simulink model "SystemModel"  (R2026a)
settings: Solver=FixedStepDiscrete  StopTime=inf  FixedStep=ts_system  EnableMultiTasking=on
StartFcn:
  | Simulink.sdi.setRecordData(false);
undefined symbols (not defined in the file): Battery, BCE12, BCE_Set_init, BMS_Controller_State, Cell10_P, Cell11_P, Cell12_P, Cell1_N, Cell1_P, Cell2_P, Cell3_P, Cell4_P, Cell5_P, Cell6_P, Cell7_P, Cell8_P, Cell9_P, Cell_Temperatures, Cell_Voltages, Charging_State, currentFactor, CV_Gain, Device_01, DiscIntNeverNeededParam, I_cc, MaxCellVoltThrsld, noCurrent, Ns_Module, NumModules, OverCellVoltageLimit, sg_bce, SOCInit, SRE, ts_controller, ts_system, UnderCellVoltageLimit, voltThreshold
libraries: slrealtimeethercatlib x99, fl_lib x65, nesl_utility x43, simulink x23, slrealtimeutilitieslib x13, sl_discontinuities x13, dspstat3 x12, canmsglib x11, speedgoatlib_IO611 x9, batt_lib x3, sharedTrackingLibrary x2, BatteryModuleLibrary_12Cells_lib x1
(part 4 of 6)

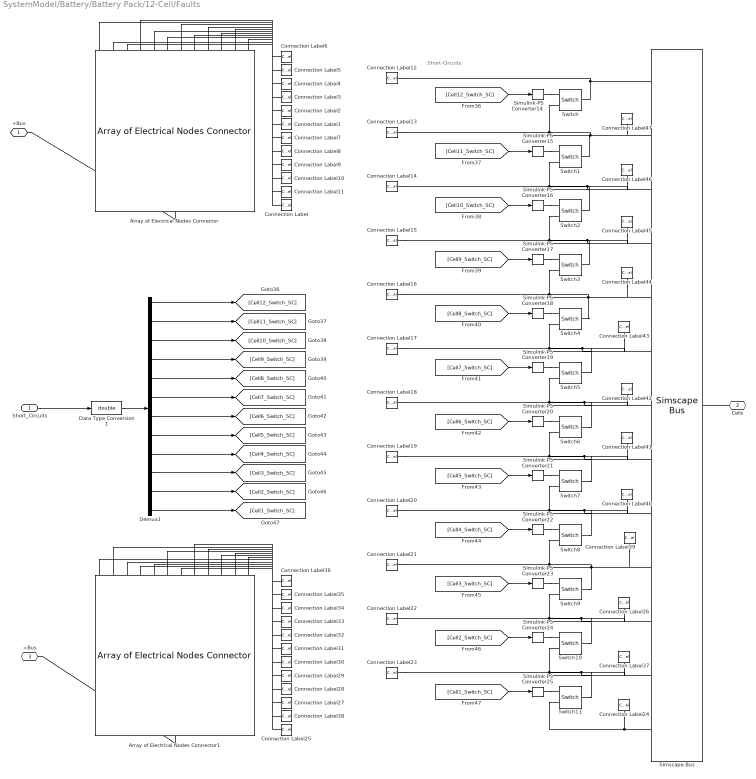
== system SystemModel/Battery/Battery Pack/12-Cell/Faults ==
  note: Short-Circuits
  Short_Circuits : Inport
  Array of Electrical Nodes Connector : batt_lib/Connectors/Array of Electrical Nodes Connector  numInputConnections=simscape.battery.enum.thermal.numArrayOfNodesConnections.twelve  inNode1NumElements=1  inNode2NumElements=1  inNode3NumElements=1  inNode4NumElements=1  inNode5NumElements=1  inNode6NumElements=1  inNode7NumElements=1  inNode8NumElements=1  inNode9NumElements=1  inNode10NumElements=1  inNode11NumElements=1  inNode12NumElements=1  inNode13NumElements=1  inNode14NumElements=1  inNode15NumElements=1  inNode16NumElements=1  inNode17NumElements=1  inNode18NumElements=1  inNode19NumElements=1  inNode20NumElements=1  inNode21NumElements=1  inNode22NumElements=1  inNode23NumElements=1  inNode24NumElements=1  inNode25NumElements=1  inNode26NumElements=1  inNode27NumElements=1  inNode28NumElements=1  inNode29NumElements=1  inNode30NumElements=1  inNode31NumElements=1  inNode32NumElements=1  inNode33NumElements=1  inNode34NumElements=1  inNode35NumElements=1  inNode36NumElements=1  inNode37NumElements=1  inNode38NumElements=1  inNode39NumElements=1  inNode40NumElements=1  inNode41NumElements=1  inNode42NumElements=1  inNode43NumElements=1  inNode44NumElements=1  inNode45NumElements=1  inNode46NumElements=1  inNode47NumElements=1  inNode48NumElements=1  inNode49NumElements=1  inNode50NumElements=1
  Array of Electrical Nodes Connector1 : batt_lib/Connectors/Array of Electrical Nodes Connector  numInputConnections=simscape.battery.enum.thermal.numArrayOfNodesConnections.twelve  inNode1NumElements=1  inNode2NumElements=1  inNode3NumElements=1  inNode4NumElements=1  inNode5NumElements=1  inNode6NumElements=1  inNode7NumElements=1  inNode8NumElements=1  inNode9NumElements=1  inNode10NumElements=1  inNode11NumElements=1  inNode12NumElements=1  inNode13NumElements=1  inNode14NumElements=1  inNode15NumElements=1  inNode16NumElements=1  inNode17NumElements=1  inNode18NumElements=1  inNode19NumElements=1  inNode20NumElements=1  inNode21NumElements=1  inNode22NumElements=1  inNode23NumElements=1  inNode24NumElements=1  inNode25NumElements=1  inNode26NumElements=1  inNode27NumElements=1  inNode28NumElements=1  inNode29NumElements=1  inNode30NumElements=1  inNode31NumElements=1  inNode32NumElements=1  inNode33NumElements=1  inNode34NumElements=1  inNode35NumElements=1  inNode36NumElements=1  inNode37NumElements=1  inNode38NumElements=1  inNode39NumElements=1  inNode40NumElements=1  inNode41NumElements=1  inNode42NumElements=1  inNode43NumElements=1  inNode44NumElements=1  inNode45NumElements=1  inNode46NumElements=1  inNode47NumElements=1  inNode48NumElements=1  inNode49NumElements=1  inNode50NumElements=1
  Connection Label : ConnectionLabel  Label=pos1
  Connection Label1 : ConnectionLabel  Label=pos7
  Connection Label10 : ConnectionLabel  Label=pos3
  Connection Label11 : ConnectionLabel  Label=pos2
  Connection Label12 : ConnectionLabel  Label=pos12
  Connection Label13 : ConnectionLabel  Label=pos11
  Connection Label14 : ConnectionLabel  Label=pos10
  Connection Label15 : ConnectionLabel  Label=pos9
  Connection Label16 : ConnectionLabel  Label=pos8
  Connection Label17 : ConnectionLabel  Label=pos7
  Connection Label18 : ConnectionLabel  Label=pos6
  Connection Label19 : ConnectionLabel  Label=pos5
  Connection Label2 : ConnectionLabel  Label=pos8
  Connection Label20 : ConnectionLabel  Label=pos4
  Connection Label21 : ConnectionLabel  Label=pos3
  Connection Label22 : ConnectionLabel  Label=pos2
  Connection Label23 : ConnectionLabel  Label=pos1
  Connection Label24 : ConnectionLabel  Label=neg1
  Connection Label25 : ConnectionLabel  Label=neg1
  Connection Label26 : ConnectionLabel  Label=neg3
  Connection Label27 : ConnectionLabel  Label=neg3
  Connection Label28 : ConnectionLabel  Label=neg4
  Connection Label29 : ConnectionLabel  Label=neg5
  Connection Label3 : ConnectionLabel  Label=pos9
  Connection Label30 : ConnectionLabel  Label=neg6
  Connection Label31 : ConnectionLabel  Label=neg7
  Connection Label32 : ConnectionLabel  Label=neg8
  Connection Label33 : ConnectionLabel  Label=neg9
  Connection Label34 : ConnectionLabel  Label=neg10
  Connection Label35 : ConnectionLabel  Label=neg11
  Connection Label36 : ConnectionLabel  Label=neg12
  Connection Label37 : ConnectionLabel  Label=neg2
  Connection Label38 : ConnectionLabel  Label=neg2
  Connection Label39 : ConnectionLabel  Label=neg4
  Connection Label4 : ConnectionLabel  Label=pos10
  Connection Label40 : ConnectionLabel  Label=neg5
  Connection Label41 : ConnectionLabel  Label=neg6
  Connection Label42 : ConnectionLabel  Label=neg7
  Connection Label43 : ConnectionLabel  Label=neg8
  Connection Label44 : ConnectionLabel  Label=neg9
  Connection Label45 : ConnectionLabel  Label=neg10
  Connection Label46 : ConnectionLabel  Label=neg11
  Connection Label47 : ConnectionLabel  Label=neg12
  Connection Label5 : ConnectionLabel  Label=pos11
  Connection Label6 : ConnectionLabel  Label=pos12
  Connection Label7 : ConnectionLabel  Label=pos6
  Connection Label8 : ConnectionLabel  Label=pos5
  Connection Label9 : ConnectionLabel  Label=pos4
  Data Type Conversion1 : DataTypeConversion  OutDataTypeStr=double  SaturateOnIntegerOverflow=off  RndMeth=Floor
  Demux1 : Demux  Outputs=12
  Simscape Bus : SimscapeBus  HierarchyStrings=Cell12_P;Cell11_P;Cell10_P;Cell9_P;Cell8_P;Cell7_P;Cell6_P;Cell5_P;Cell4_P;Cell3_P;Cell2_P;Cell1_P;Cell1_N
  Simulink-PS Converter{14..25} (12 alike) : nesl_utility/Simulink-PS Converter  PhysicalDomain=network_engine_domain  SubClassName=ps_input  LeftPortType=input  RightPortType=output  PseudoPeriodic=off  Frequencies=[]  NoiseDistribution=none  NoiseParameters=[]  Unit=1  AffineConversion=off  FilteringAndDerivatives=zero  SimscapeFilterOrder=1  InputFilterTimeConstant=0.001  UdotUserProvided=1
  Switch{,1..11} (12 alike) : fl_lib/Electrical/Electrical Elements/Switch  R_closed=0.01 Ohm  G_open=1e-8 1/Ohm  Threshold=0.5  i_specify=off  i_priority=None  i=0 A  i_nominal_specify=off  i_nominal_value=1  i_nominal_unit=A  v_specify=off  v_priority=None  v=0 V  v_nominal_specify=off  v_nominal_value=1  v_nominal_unit=V
  +Bus : PMIOPort  Side=Right
  Cells : PMIOPort  Port=2  Side=Right
  =Bus : PMIOPort  Port=3  Side=Right
  wires:
  [Cell2_Switch_SC] -> Simulink-PS Converter24/1
  [Cell3_Switch_SC] -> Simulink-PS Converter23/1
  Demux1/9 -> [Cell4_Switch_SC]
  Data Type Conversion1/1 -> Demux1/1
  Demux1/5 -> [Cell8_Switch_SC]
  Demux1/8 -> [Cell5_Switch_SC]
  [Cell1_Switch_SC] -> Simulink-PS Converter25/1
  [Cell12_Switch_SC] -> Simulink-PS Converter14/1
  [Cell11_Switch_SC] -> Simulink-PS Converter15/1
  Demux1/1 -> [Cell12_Switch_SC]
  Demux1/7 -> [Cell6_Switch_SC]
  [Cell4_Switch_SC] -> Simulink-PS Converter22/1
  Demux1/10 -> [Cell3_Switch_SC]
  Demux1/2 -> [Cell11_Switch_SC]
  [Cell8_Switch_SC] -> Simulink-PS Converter18/1
  [Cell5_Switch_SC] -> Simulink-PS Converter21/1
  Demux1/12 -> [Cell1_Switch_SC]
  [Cell10_Switch_SC] -> Simulink-PS Converter16/1
  [Cell9_Switch_SC] -> Simulink-PS Converter17/1
  Demux1/3 -> [Cell10_Switch_SC]
  Demux1/6 -> [Cell7_Switch_SC]
  [Cell6_Switch_SC] -> Simulink-PS Converter20/1
  [Cell7_Switch_SC] -> Simulink-PS Converter19/1
  Demux1/4 -> [Cell9_Switch_SC]
  Demux1/11 -> [Cell2_Switch_SC]
  Short_Circuits/1 -> Data Type Conversion1/1
  connections:
  Simulink-PS Converter17/RConn1 -- Switch3/RConn1
  Connection Label10/LConn1 -- Array of Electrical Nodes Connector/LConn10
  Switch3/LConn1 -- Connection Label45/LConn1 -- Simscape Bus/LConn4 -- Connection Label15/LConn1 -- Switch2/RConn2
  Switch6/LConn1 -- Connection Label42/LConn1 -- Simscape Bus/LConn7 -- Connection Label18/LConn1 -- Switch5/RConn2
  Connection Label31/LConn1 -- Array of Electrical Nodes Connector1/LConn6
  Switch7/LConn1 -- Connection Label41/LConn1 -- Simscape Bus/LConn8 -- Connection Label19/LConn1 -- Switch6/RConn2
  Switch2/LConn1 -- Connection Label46/LConn1 -- Simscape Bus/LConn3 -- Connection Label14/LConn1 -- Switch1/RConn2
  Connection Label28/LConn1 -- Array of Electrical Nodes Connector1/LConn9
  Connection Label29/LConn1 -- Array of Electrical Nodes Connector1/LConn8
  Simulink-PS Converter16/RConn1 -- Switch2/RConn1
  Simulink-PS Converter19/RConn1 -- Switch5/RConn1
  Switch10/LConn1 -- Connection Label26/LConn1 -- Simscape Bus/LConn11 -- Connection Label22/LConn1 -- Switch9/RConn2
  Simulink-PS Converter25/RConn1 -- Switch11/RConn1
  Connection Label27/LConn1 -- Array of Electrical Nodes Connector1/LConn10
  Connection Label25/LConn1 -- Array of Electrical Nodes Connector1/LConn12
  Switch11/LConn1 -- Connection Label37/LConn1 -- Simscape Bus/LConn12 -- Connection Label23/LConn1 -- Switch10/RConn2
  Connection Label39/LConn1 -- Simscape Bus/LConn10 -- Switch9/LConn1 -- Connection Label21/LConn1 -- Switch8/RConn2
  Connection Label36/LConn1 -- Array of Electrical Nodes Connector1/LConn1
  Connection Label34/LConn1 -- Array of Electrical Nodes Connector1/LConn3
  Connection Label35/LConn1 -- Array of Electrical Nodes Connector1/LConn2
  Simulink-PS Converter14/RConn1 -- Switch/RConn1
  Simscape Bus/LConn13 -- Connection Label24/LConn1 -- Switch11/RConn2
  Connection Label30/LConn1 -- Array of Electrical Nodes Connector1/LConn7
  Simulink-PS Converter18/RConn1 -- Switch4/RConn1
  Connection Label44/LConn1 -- Simscape Bus/LConn5 -- Switch4/LConn1 -- Connection Label16/LConn1 -- Switch3/RConn2
  Simulink-PS Converter24/RConn1 -- Switch10/RConn1
  Connection Label33/LConn1 -- Array of Electrical Nodes Connector1/LConn4
  Connection Label38/LConn1 -- Array of Electrical Nodes Connector1/LConn11
  Connection Label32/LConn1 -- Array of Electrical Nodes Connector1/LConn5
  Switch8/LConn1 -- Connection Label40/LConn1 -- Simscape Bus/LConn9 -- Connection Label20/LConn1 -- Switch7/RConn2
  Cells/RConn1 -- Simscape Bus/RConn1
  Simulink-PS Converter20/RConn1 -- Switch6/RConn1
  Simulink-PS Converter15/RConn1 -- Switch1/RConn1
  Simulink-PS Converter21/RConn1 -- Switch7/RConn1
  Simulink-PS Converter23/RConn1 -- Switch9/RConn1
  Simulink-PS Converter22/RConn1 -- Switch8/RConn1
  Connection Label11/LConn1 -- Array of Electrical Nodes Connector/LConn11
  Connection Label6/LConn1 -- Array of Electrical Nodes Connector/LConn1
  Connection Label7/LConn1 -- Array of Electrical Nodes Connector/LConn7
  Switch5/LConn1 -- Connection Label43/LConn1 -- Simscape Bus/LConn6 -- Connection Label17/LConn1 -- Switch4/RConn2
  Connection Label2/LConn1 -- Array of Electrical Nodes Connector/LConn5
  Simscape Bus/LConn1 -- Connection Label12/LConn1 -- Switch/LConn1
  Connection Label4/LConn1 -- Array of Electrical Nodes Connector/LConn3
  Connection Label8/LConn1 -- Array of Electrical Nodes Connector/LConn8
  Connection Label5/LConn1 -- Array of Electrical Nodes Connector/LConn2
  Connection Label3/LConn1 -- Array of Electrical Nodes Connector/LConn4
  Connection Label1/LConn1 -- Array of Electrical Nodes Connector/LConn6
  Connection Label/LConn1 -- Array of Electrical Nodes Connector/LConn12
  Connection Label9/LConn1 -- Array of Electrical Nodes Connector/LConn9
  Connection Label47/LConn1 -- Simscape Bus/LConn2 -- Switch1/LConn1 -- Connection Label13/LConn1 -- Switch/RConn2
  Array of Electrical Nodes Connector1/RConn1 -- =Bus/RConn1
  Array of Electrical Nodes Connector/RConn1 -- +Bus/RConn1

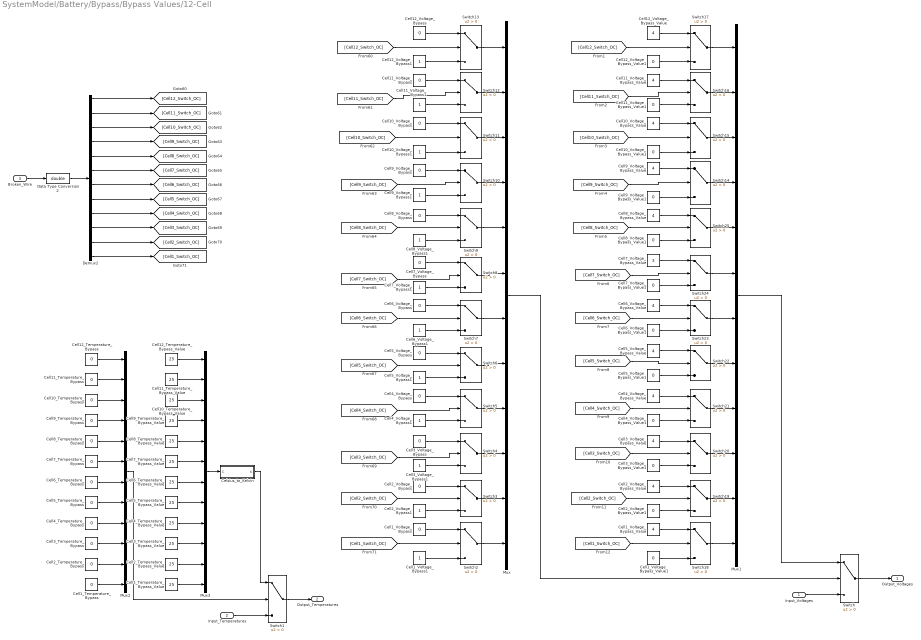
== system SystemModel/Battery/Bypass/Bypass Values/12-Cell ==
  Input_Voltages : Inport
  Input_Temperatures : Inport  Port=2
  Broken_Wire : Inport  Port=3
  Cell10_Temperature_Bypass : Constant  Value=0  SampleTime=-1
  Cell10_Temperature_Bypass_Value : Constant  Value=25  SampleTime=-1
  Cell10_Voltage_Bypass : Constant  Value=0  SampleTime=-1
  Cell10_Voltage_Bypass1 : Constant  SampleTime=-1
  Cell10_Voltage_Bypass_Value : Constant  Value=4  SampleTime=-1
  Cell10_Voltage_Bypass_Value1 : Constant  Value=0  SampleTime=-1
  Cell11_Temperature_Bypass : Constant  Value=0  SampleTime=-1
  Cell11_Temperature_Bypass_Value : Constant  Value=25  SampleTime=-1
  Cell11_Voltage_Bypass : Constant  Value=0  SampleTime=-1
  Cell11_Voltage_Bypass1 : Constant  SampleTime=-1
  Cell11_Voltage_Bypass_Value : Constant  Value=4  SampleTime=-1
  Cell11_Voltage_Bypass_Value1 : Constant  Value=0  SampleTime=-1
  Cell12_Temperature_Bypass : Constant  Value=0  SampleTime=-1
  Cell12_Temperature_Bypass_Value : Constant  Value=25  SampleTime=-1
  Cell12_Voltage_Bypass : Constant  Value=0  SampleTime=-1
  Cell12_Voltage_Bypass1 : Constant  SampleTime=-1
  Cell12_Voltage_Bypass_Value : Constant  Value=4  SampleTime=-1
  Cell12_Voltage_Bypass_Value1 : Constant  Value=0  SampleTime=-1
  Cell1_Temperature_Bypass : Constant  Value=0  SampleTime=-1
  Cell1_Temperature_Bypass_Value : Constant  Value=25  SampleTime=-1
  Cell1_Voltage_Bypass : Constant  Value=0  SampleTime=-1
  Cell1_Voltage_Bypass1 : Constant  SampleTime=-1
  Cell1_Voltage_Bypass_Value : Constant  Value=4  SampleTime=-1
  Cell1_Voltage_Bypass_Value1 : Constant  Value=0  SampleTime=-1
  Cell2_Temperature_Bypass : Constant  Value=0  SampleTime=-1
  Cell2_Temperature_Bypass_Value : Constant  Value=25  SampleTime=-1
  Cell2_Voltage_Bypass : Constant  Value=0  SampleTime=-1
  Cell2_Voltage_Bypass1 : Constant  SampleTime=-1
  Cell2_Voltage_Bypass_Value : Constant  Value=4  SampleTime=-1
  Cell2_Voltage_Bypass_Value1 : Constant  Value=0  SampleTime=-1
  Cell3_Temperature_Bypass : Constant  Value=0  SampleTime=-1
  Cell3_Temperature_Bypass_Value : Constant  Value=25  SampleTime=-1
  Cell3_Voltage_Bypass : Constant  Value=0  SampleTime=-1
  Cell3_Voltage_Bypass1 : Constant  SampleTime=-1
  Cell3_Voltage_Bypass_Value : Constant  Value=4  SampleTime=-1
  Cell3_Voltage_Bypass_Value1 : Constant  Value=0  SampleTime=-1
  Cell4_Temperature_Bypass : Constant  Value=0  SampleTime=-1
  Cell4_Temperature_Bypass_Value : Constant  Value=25  SampleTime=-1
  Cell4_Voltage_Bypass : Constant  Value=0  SampleTime=-1
  Cell4_Voltage_Bypass1 : Constant  SampleTime=-1
  Cell4_Voltage_Bypass_Value : Constant  Value=4  SampleTime=-1
  Cell4_Voltage_Bypass_Value1 : Constant  Value=0  SampleTime=-1
  Cell5_Temperature_Bypass : Constant  Value=0  SampleTime=-1
  Cell5_Temperature_Bypass_Value : Constant  Value=25  SampleTime=-1
  Cell5_Voltage_Bypass : Constant  Value=0  SampleTime=-1
  Cell5_Voltage_Bypass1 : Constant  SampleTime=-1
  Cell5_Voltage_Bypass_Value : Constant  Value=4  SampleTime=-1
  Cell5_Voltage_Bypass_Value1 : Constant  Value=0  SampleTime=-1
  Cell6_Temperature_Bypass : Constant  Value=0  SampleTime=-1
  Cell6_Temperature_Bypass_Value : Constant  Value=25  SampleTime=-1
  Cell6_Voltage_Bypass : Constant  Value=0  SampleTime=-1
  Cell6_Voltage_Bypass1 : Constant  SampleTime=-1
  Cell6_Voltage_Bypass_Value : Constant  Value=4  SampleTime=-1
  Cell6_Voltage_Bypass_Value1 : Constant  Value=0  SampleTime=-1
  Cell7_Temperature_Bypass : Constant  Value=0  SampleTime=-1
  Cell7_Temperature_Bypass_Value : Constant  Value=25  SampleTime=-1
  Cell7_Voltage_Bypass : Constant  Value=0  SampleTime=-1
  Cell7_Voltage_Bypass1 : Constant  SampleTime=-1
  Cell7_Voltage_Bypass_Value : Constant  Value=3  SampleTime=-1
  Cell7_Voltage_Bypass_Value1 : Constant  Value=0  SampleTime=-1
  Cell8_Temperature_Bypass : Constant  Value=0  SampleTime=-1
  Cell8_Temperature_Bypass_Value : Constant  Value=25  SampleTime=-1
  Cell8_Voltage_Bypass : Constant  Value=0  SampleTime=-1
  Cell8_Voltage_Bypass1 : Constant  SampleTime=-1
  Cell8_Voltage_Bypass_Value : Constant  Value=4  SampleTime=-1
  Cell8_Voltage_Bypass_Value1 : Constant  Value=0  SampleTime=-1
  Cell9_Temperature_Bypass : Constant  Value=0  SampleTime=-1
  Cell9_Temperature_Bypass_Value : Constant  Value=25  SampleTime=-1
  Cell9_Voltage_Bypass : Constant  Value=0  SampleTime=-1
  Cell9_Voltage_Bypass1 : Constant  SampleTime=-1
  Cell9_Voltage_Bypass_Value : Constant  Value=4  SampleTime=-1
  Cell9_Voltage_Bypass_Value1 : Constant  Value=0  SampleTime=-1
  Celsius_to_Kelvin : Subsystem
  Data Type Conversion2 : DataTypeConversion  OutDataTypeStr=double  SaturateOnIntegerOverflow=off  RndMeth=Floor
  Demux2 : Demux  Outputs=12
  Mux{,1..3} (4 alike) : Mux  Inputs=12
  Switch{,1..25} (26 alike) : Switch  Criteria=u2 > Threshold  SaturateOnIntegerOverflow=off  InputSameDT=off
  Output_Voltages : Outport
  Output_Temperatures : Outport  Port=2
  wires:
  Mux/1 -> Switch/2
  Switch/1 -> Output_Voltages/1
  Mux1/1 -> Switch/1
  Input_Voltages/1 -> Switch/3
  Cell11_Temperature_Bypass/1 -> Mux2/2
  Cell1_Temperature_Bypass/1 -> Mux2/12
  Cell5_Temperature_Bypass/1 -> Mux2/8
  Cell6_Temperature_Bypass/1 -> Mux2/7
  Cell10_Temperature_Bypass/1 -> Mux2/3
  Cell4_Temperature_Bypass/1 -> Mux2/9
  Cell2_Temperature_Bypass/1 -> Mux2/11
  Cell9_Temperature_Bypass/1 -> Mux2/4
  Cell8_Temperature_Bypass_Value/1 -> Mux3/5
  Cell10_Temperature_Bypass_Value/1 -> Mux3/3
  Mux3/1 -> Celsius_to_Kelvin/1(C)
  Cell12_Temperature_Bypass_Value/1 -> Mux3/1
  Cell1_Temperature_Bypass_Value/1 -> Mux3/12
  Cell11_Temperature_Bypass_Value/1 -> Mux3/2
  Cell8_Temperature_Bypass/1 -> Mux2/5
  Cell3_Temperature_Bypass_Value/1 -> Mux3/10
  Cell9_Temperature_Bypass_Value/1 -> Mux3/4
  Cell6_Temperature_Bypass_Value/1 -> Mux3/7
  Cell12_Temperature_Bypass/1 -> Mux2/1
  Cell5_Temperature_Bypass_Value/1 -> Mux3/8
  Cell2_Temperature_Bypass_Value/1 -> Mux3/11
  Cell7_Temperature_Bypass/1 -> Mux2/6
  Mux2/1 -> Switch1/2
  Celsius_to_Kelvin/1(K) -> Switch1/1
  Cell4_Temperature_Bypass_Value/1 -> Mux3/9
  Input_Temperatures/1 -> Switch1/3
  Cell3_Temperature_Bypass/1 -> Mux2/10
  Cell7_Temperature_Bypass_Value/1 -> Mux3/6
  Switch1/1 -> Output_Temperatures/1
  Switch2/1 -> Mux/12
  [Cell5_Switch_OC] -> Switch6/2
  [Cell1_Switch_OC] -> Switch2/2
  [Cell8_Switch_OC] -> Switch9/2
  [Cell6_Switch_OC] -> Switch7/2
  [Cell7_Switch_OC] -> Switch8/2
  [Cell10_Switch_OC] -> Switch11/2
  [Cell12_Switch_OC] -> Switch13/2
  [Cell3_Switch_OC] -> Switch4/2
  [Cell9_Switch_OC] -> Switch10/2
  [Cell4_Switch_OC] -> Switch5/2
  [Cell11_Switch_OC] -> Switch12/2
  [Cell2_Switch_OC] -> Switch3/2
  Switch3/1 -> Mux/11
  Switch13/1 -> Mux/1
  Switch12/1 -> Mux/2
  Switch11/1 -> Mux/3
  Switch10/1 -> Mux/4
  Switch9/1 -> Mux/5
  Switch8/1 -> Mux/6
  Switch7/1 -> Mux/7
  Switch6/1 -> Mux/8
  Switch5/1 -> Mux/9
  Switch4/1 -> Mux/10
  Cell1_Voltage_Bypass/1 -> Switch2/1
  Cell2_Voltage_Bypass/1 -> Switch3/1
  Cell12_Voltage_Bypass/1 -> Switch13/1
  Cell11_Voltage_Bypass/1 -> Switch12/1
  Cell10_Voltage_Bypass/1 -> Switch11/1
  Cell9_Voltage_Bypass/1 -> Switch10/1
  Cell8_Voltage_Bypass/1 -> Switch9/1
  Cell7_Voltage_Bypass/1 -> Switch8/1
  Cell6_Voltage_Bypass/1 -> Switch7/1
  Cell5_Voltage_Bypass/1 -> Switch6/1
  Cell4_Voltage_Bypass/1 -> Switch5/1
  Cell3_Voltage_Bypass/1 -> Switch4/1
  Cell1_Voltage_Bypass1/1 -> Switch2/3
  Cell2_Voltage_Bypass1/1 -> Switch3/3
  Cell3_Voltage_Bypass1/1 -> Switch4/3
  Cell4_Voltage_Bypass1/1 -> Switch5/3
  Cell5_Voltage_Bypass1/1 -> Switch6/3
  Cell6_Voltage_Bypass1/1 -> Switch7/3
  Cell7_Voltage_Bypass1/1 -> Switch8/3
  Cell8_Voltage_Bypass1/1 -> Switch9/3
  Cell9_Voltage_Bypass1/1 -> Switch10/3
  Cell10_Voltage_Bypass1/1 -> Switch11/3
  Cell11_Voltage_Bypass1/1 -> Switch12/3
  Cell12_Voltage_Bypass1/1 -> Switch13/3
  Switch17/1 -> Mux1/1
  Switch16/1 -> Mux1/2
  Switch18/1 -> Mux1/12
  Switch25/1 -> Mux1/5
  Switch20/1 -> Mux1/10
  Switch19/1 -> Mux1/11
  Switch15/1 -> Mux1/3
  Switch14/1 -> Mux1/4
  Switch24/1 -> Mux1/6
  Switch23/1 -> Mux1/7
  Switch22/1 -> Mux1/8
  Switch21/1 -> Mux1/9
  Cell12_Voltage_Bypass_Value/1 -> Switch17/1
  Cell11_Voltage_Bypass_Value/1 -> Switch16/1
  Cell10_Voltage_Bypass_Value/1 -> Switch15/1
  Cell9_Voltage_Bypass_Value/1 -> Switch14/1
  Cell8_Voltage_Bypass_Value/1 -> Switch25/1
  Cell6_Voltage_Bypass_Value/1 -> Switch23/1
  Cell5_Voltage_Bypass_Value/1 -> Switch22/1
  Cell4_Voltage_Bypass_Value/1 -> Switch21/1
  Cell3_Voltage_Bypass_Value/1 -> Switch20/1
  Cell2_Voltage_Bypass_Value/1 -> Switch19/1
  Cell1_Voltage_Bypass_Value/1 -> Switch18/1
  Cell7_Voltage_Bypass_Value/1 -> Switch24/1
  Cell12_Voltage_Bypass_Value1/1 -> Switch17/3
  Cell11_Voltage_Bypass_Value1/1 -> Switch16/3
  Cell10_Voltage_Bypass_Value1/1 -> Switch15/3
  Cell9_Voltage_Bypass_Value1/1 -> Switch14/3
  Cell8_Voltage_Bypass_Value1/1 -> Switch25/3
  Cell7_Voltage_Bypass_Value1/1 -> Switch24/3
  Cell6_Voltage_Bypass_Value1/1 -> Switch23/3
  Cell5_Voltage_Bypass_Value1/1 -> Switch22/3
  Cell4_Voltage_Bypass_Value1/1 -> Switch21/3
  Cell3_Voltage_Bypass_Value1/1 -> Switch20/3
  Cell2_Voltage_Bypass_Value1/1 -> Switch19/3
  Cell1_Voltage_Bypass_Value1/1 -> Switch18/3
  [Cell12_Switch_OC] -> Switch17/2
  [Cell10_Switch_OC] -> Switch15/2
  [Cell11_Switch_OC] -> Switch16/2
  [Cell9_Switch_OC] -> Switch14/2
  [Cell8_Switch_OC] -> Switch25/2
  [Cell7_Switch_OC] -> Switch24/2
  [Cell6_Switch_OC] -> Switch23/2
  [Cell5_Switch_OC] -> Switch22/2
  [Cell4_Switch_OC] -> Switch21/2
  [Cell3_Switch_OC] -> Switch20/2
  [Cell2_Switch_OC] -> Switch19/2
  [Cell1_Switch_OC] -> Switch18/2
  Demux2/6 -> [Cell7_Switch_OC]
  Demux2/12 -> [Cell1_Switch_OC]
  Broken_Wire/1 -> Data Type Conversion2/1
  Demux2/5 -> [Cell8_Switch_OC]
  Demux2/11 -> [Cell2_Switch_OC]
  Demux2/7 -> [Cell6_Switch_OC]
  Demux2/3 -> [Cell10_Switch_OC]
  Demux2/9 -> [Cell4_Switch_OC]
  Demux2/2 -> [Cell11_Switch_OC]
  Demux2/10 -> [Cell3_Switch_OC]
  Demux2/4 -> [Cell9_Switch_OC]
  Demux2/8 -> [Cell5_Switch_OC]
  Data Type Conversion2/1 -> Demux2/1
  Demux2/1 -> [Cell12_Switch_OC]

== system SystemModel/Battery/HW Interface/BCE - HIL/Battery Cell Emulator ==
  Sensor_Values_Sim : Inport
  "BCE Bus Packing " : Subsystem
  "BCE Read " : Subsystem  InitFcn=sg_bce.checkNumberOfBlocksGlobal(bdroot);  mask(bce_read){}
      settings: OpenFcn=sg_bce.openFcnRead;
      mask Help: eval('sg.utils.help.show(''io_main/refentry_bce_read'');')
      mask Display: disp('Speedgoat\nBMTS Read\nEtherCAT Bus: 0, Device: 1\nBCE12-0505');port_label('output',1,'Data');
  "BCE Setup " : Subsystem  LoadFcn=|  InitFcn=|  mask(bce_setup){}
      LoadFcn=|
      | sg_bce.createBusSignals;
      | sg_bce.setupEniCallback(gcb, bdroot);
      InitFcn=|
      | sg_bce.createBusSignals;
      | sg_bce.checkNumberOfBlocksGlobal(bdroot);
      mask init:
      | sg_bce.setupEniCallback(gcb, bdroot);
      settings: OpenFcn=sg_bce.openFcnSetup;
      mask Help: eval('sg.utils.help.show(''io_main/refentry_bce_setup'');')
      mask Display: disp('Speedgoat\nBattery Management Testing Systems\nEtherCAT Bus: 0\nSetup');
  "BCE Write " : Subsystem  InitFcn=sg_bce.checkNumberOfBlocksGlobal(bdroot);  mask(bce_write){}
      settings: OpenFcn=sg_bce.openFcnWrite;
      mask Help: eval('sg.utils.help.show(''io_main/refentry_bce_write'');')
      mask Display: disp('Speedgoat\nBMTS Write\nEtherCAT Bus: 0, Device: 1\nBCE12-0505');port_label('input',1,'Data');
  BCE_Init : Switch  Criteria=u2 > Threshold  SaturateOnIntegerOverflow=off  InputSameDT=off
  Bus Selector : BusSelector  OutputSignals=Cell_12.I,Cell_11.I,Cell_10.I,Cell_9.I,Cell_8.I,Cell_7.I,Cell_6.I,Cell_5.I,Cell_4.I,Cell_3.I,Cell_2.I,Cell_1.I
  Bus Selector1 : BusSelector  OutputSignals=Cell_Voltages
  Bus Selector2 : BusSelector  OutputSignals=Cell_12.V,Cell_11.V,Cell_10.V,Cell_9.V,Cell_8.V,Cell_7.V,Cell_6.V,Cell_5.V,Cell_4.V,Cell_3.V,Cell_2.V,Cell_1.V
  Constant : Constant  Value=[0,0,0,0,0,0,0,0,0,0,0,0]
  Data Type Conversion : DataTypeConversion  OutDataTypeStr=single  SaturateOnIntegerOverflow=off  RndMeth=Floor
  Data Type Conversion1 : DataTypeConversion  OutDataTypeStr=boolean  SaturateOnIntegerOverflow=off  RndMeth=Floor
  Data Type Conversion2 : DataTypeConversion  OutDataTypeStr=single  SaturateOnIntegerOverflow=off  RndMeth=Floor
  Demux : Demux  Outputs=12
  Enable : Constant
  Mux : Mux  Inputs=12
  Mux1 : Mux  Inputs=12
  No_current : Constant  Value=0
  Step : Step  Time=2
  Current_Values : Outport
  Cell_Voltages : Outport  Port=2
  wires:
  Sensor_Values_Sim/1 -> Bus Selector1/1
  BCE_Init/1 -> Demux/1
  "BCE Read "/1(Data) -> Bus Selector/1, Bus Selector2/1
  Constant/1 -> Data Type Conversion2/1
  Step/1 -> BCE_Init/2
  "BCE Bus Packing "/1(BCE Bus) -> "BCE Write "/1(Data)
  No_current/1 -> Data Type Conversion/1
  Data Type Conversion2/1 -> BCE_Init/3
  Bus Selector/1 -> Mux/1  "<I>"
  Bus Selector/2 -> Mux/2  "<I>"
  Bus Selector/3 -> Mux/3  "<I>"
  Bus Selector/4 -> Mux/4  "<I>"
  Bus Selector/5 -> Mux/5  "<I>"
  Bus Selector/6 -> Mux/6  "<I>"
  Bus Selector/7 -> Mux/7  "<I>"
  Bus Selector/8 -> Mux/8  "<I>"
  Bus Selector/9 -> Mux/9  "<I>"
  Bus Selector/10 -> Mux/10  "<I>"
  Bus Selector/11 -> Mux/11  "<I>"
  Bus Selector/12 -> Mux/12  "<I>"
  Mux/1 -> Current_Values/1
  Bus Selector2/1 -> Mux1/1  "<V>"
  Bus Selector2/2 -> Mux1/2  "<V>"
  Bus Selector2/3 -> Mux1/3  "<V>"
  Bus Selector2/4 -> Mux1/4  "<V>"
  Bus Selector2/5 -> Mux1/5  "<V>"
  Bus Selector2/6 -> Mux1/6  "<V>"
  Bus Selector2/7 -> Mux1/7  "<V>"
  Bus Selector2/8 -> Mux1/8  "<V>"
  Bus Selector2/9 -> Mux1/9  "<V>"
  Bus Selector2/10 -> Mux1/10  "<V>"
  Bus Selector2/11 -> Mux1/11  "<V>"
  Bus Selector2/12 -> Mux1/12  "<V>"
  Mux1/1 -> Cell_Voltages/1
  Bus Selector1/1 -> BCE_Init/1  "<Cell_Voltages>"
  Enable/1 -> Data Type Conversion1/1
  Data Type Conversion1/1 -> "BCE Bus Packing "/1(Cell 1 Enable), "BCE Bus Packing "/9(Cell 9 Enable), "BCE Bus Packing "/12(Cell 12 Enable), "BCE Bus Packing "/11(Cell 11 Enable), "BCE Bus Packing "/10(Cell 10 Enable), "BCE Bus Packing "/8(Cell 8 Enable), "BCE Bus Packing "/7(Cell 7 Enable), "BCE Bus Packing "/6(Cell 6 Enable), "BCE Bus Packing "/5(Cell 5 Enable), "BCE Bus Packing "/4(Cell 4 Enable), "BCE Bus Packing "/3(Cell 3 Enable), "BCE Bus Packing "/2(Cell 2 Enable)
  Data Type Conversion/1 -> "BCE Bus Packing "/29(Cell 5 Current), "BCE Bus Packing "/28(Cell 4 Current), "BCE Bus Packing "/25(Cell 1 Current), "BCE Bus Packing "/26(Cell 2 Current), "BCE Bus Packing "/27(Cell 3 Current), "BCE Bus Packing "/30(Cell 6 Current), "BCE Bus Packing "/31(Cell 7 Current), "BCE Bus Packing "/32(Cell 8 Current), "BCE Bus Packing "/33(Cell 9 Current), "BCE Bus Packing "/34(Cell 10 Current), "BCE Bus Packing "/35(Cell 11 Current), "BCE Bus Packing "/36(Cell 12 Current)
  Demux/1 -> "BCE Bus Packing "/13(Cell 12 Voltage)
  Demux/2 -> "BCE Bus Packing "/14(Cell 11 Voltage)
  Demux/3 -> "BCE Bus Packing "/15(Cell 10 Voltage)
  Demux/4 -> "BCE Bus Packing "/16(Cell 9 Voltage)
  Demux/5 -> "BCE Bus Packing "/17(Cell 8 Voltage)
  Demux/6 -> "BCE Bus Packing "/18(Cell 7 Voltage)
  Demux/7 -> "BCE Bus Packing "/19(Cell 6 Voltage)
  Demux/8 -> "BCE Bus Packing "/20(Cell 5 Voltage)
  Demux/9 -> "BCE Bus Packing "/21(Cell 4 Voltage)
  Demux/10 -> "BCE Bus Packing "/22(Cell 3 Voltage)
  Demux/11 -> "BCE Bus Packing "/23(Cell 2 Voltage)
  Demux/12 -> "BCE Bus Packing "/24(Cell 1 Voltage)

== system SystemModel/Battery/HW Interface/BCE - HIL/Shunt Emulator ==
  note: Shunt Emulator Blocks
  Sensor_Values_Sim : Inport
  Bus Selector : BusSelector  OutputSignals=Pack_Current
  Pack_Current : Outport
  wires:
  Sensor_Values_Sim/1 -> Bus Selector/1
  Bus Selector/1 -> Pack_Current/1  "<Pack_Current>"

== system SystemModel/Battery/HW Interface/BCE - HIL/Temperature Emulator ==
  note: Temperature Emulation Blocks
  Sensor_Values_Sim : Inport
  Bus Selector : BusSelector  OutputSignals=Cell_Temperatures
  Cell_Temperatures : Outport
  wires:
  Sensor_Values_Sim/1 -> Bus Selector/1
  Bus Selector/1 -> Cell_Temperatures/1  "<Cell_Temperatures>"

== system SystemModel/Instrumentation/Instrumented Signals/12-Cell/Celsius_to_Kelvin ==
  K : Inport
  Add : Sum  Inputs=+-
  Constant4 : Constant  Value=273.15
  C : Outport
  wires:
  Constant4/1 -> Add/2
  K/1 -> Add/1
  Add/1 -> C/1

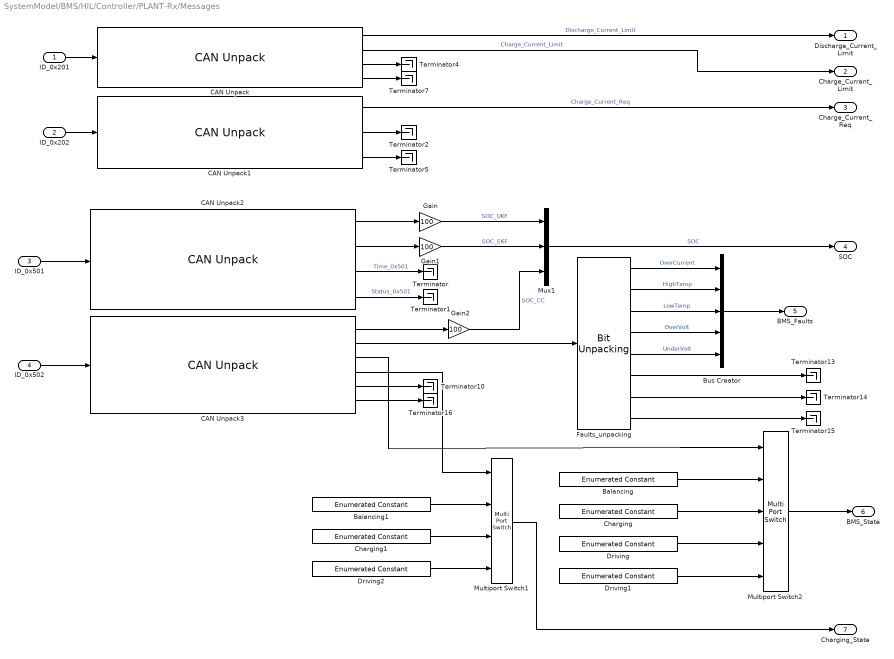
== system SystemModel/BMS/HIL/Controller/PLANT-Rx/Messages ==
  ID_0x201 : Inport
  ID_0x202 : Inport  Port=2
  ID_0x501 : Inport  Port=3
  ID_0x502 : Inport  Port=4
  Balancing : simulink/Sources/Enumerated Constant  OutDataTypeStr=Enum: BMS_Controller_State  Value=BMS_Controller_State.BMS_Idle  SampleTime=-1
  Balancing1 : simulink/Sources/Enumerated Constant  OutDataTypeStr=Enum: Charging_State  Value=Charging_State.Init  SampleTime=-1
  Bus Creator : BusCreator  Inputs=5  OutDataTypeStr=Bus: Faults
  CAN Unpack : canmsglib/CAN Unpack  MsgList=(none)  MsgName=CAN Msg  MsgIDType=Standard (11-bit identifier)  MsgIdentifier=0x201  MsgLength=8  SignalInfo={ 'DischargeCurrentLimit_CAN', '0', '32', 'LE', 'single', 'Standard', '0', '1', '0', '-inf', '+inf'; 'ChargeCurrentLimit_CAN', '32', '32', 'LE', 'single', 'Standard', '0', '1', '0', '-Inf', 'Inf' }  IDPort=off  TimestampPort=on  ErrorPort=off  RemotePort=off  LengthPort=off  StatusPort=on  ApplyMinMax=off
      settings: LibrarySourceBlock=embeddedtargetslib/Host Communication/CAN Unpack
  CAN Unpack1 : canmsglib/CAN Unpack  MsgList=(none)  MsgName=CAN Msg  MsgIDType=Standard (11-bit identifier)  MsgIdentifier=0x202  MsgLength=4  SignalInfo={ 'ChargeCurrentReq', '0', '32', 'LE', 'single', 'Standard', '0', '1', '0', '-inf', '+inf' }  IDPort=off  TimestampPort=on  ErrorPort=off  RemotePort=off  LengthPort=off  StatusPort=on  ApplyMinMax=off
      settings: LibrarySourceBlock=embeddedtargetslib/Host Communication/CAN Unpack
  CAN Unpack2 : canmsglib/CAN Unpack  MsgList=(none)  MsgName=CAN Msg  MsgIDType=Standard (11-bit identifier)  MsgIdentifier=0x501  MsgLength=8  SignalInfo={ 'SOC_UKF', '0', '32', 'LE', 'single', 'Standard', '0', '1', '0', '-inf', '+inf'; 'SOC_EKF', '32', '32', 'LE', 'single', 'Standard', '0', '1', '0', '-Inf', 'Inf' }  IDPort=off  TimestampPort=on  ErrorPort=off  RemotePort=off  LengthPort=off  StatusPort=on  ApplyMinMax=off
      settings: LibrarySourceBlock=embeddedtargetslib/Host Communication/CAN Unpack
  CAN Unpack3 : canmsglib/CAN Unpack  MsgList=(none)  MsgName=CAN Msg  MsgIDType=Standard (11-bit identifier)  MsgIdentifier=0x502  MsgLength=7  SignalInfo={ 'SOC_CC', '0', '32', 'LE', 'single', 'Standard', '0', '1', '0', '-inf', '+inf'; 'Faults', '32', '8', 'LE', 'unsigned', 'Standard', '0', '1', '0', '-Inf', 'Inf'; 'BMS_State', '40', '8', 'LE', 'unsigned', 'Standard', '0', '1', '0', '-Inf', 'Inf'; 'Charging_State', '48', '8', 'LE', 'signed', 'Standard', '0', '1', '0', '-Inf', 'Inf' }  IDPort=off  TimestampPort=on  ErrorPort=off  RemotePort=off  LengthPort=off  StatusPort=on  ApplyMinMax=off
      settings: LibrarySourceBlock=embeddedtargetslib/Host Communication/CAN Unpack
  Charging : simulink/Sources/Enumerated Constant  OutDataTypeStr=Enum: BMS_Controller_State  Value=BMS_Controller_State.BMS_Driving  SampleTime=-1
  Charging1 : simulink/Sources/Enumerated Constant  OutDataTypeStr=Enum: Charging_State  Value=Charging_State.CC  SampleTime=-1
  Driving : simulink/Sources/Enumerated Constant  OutDataTypeStr=Enum: BMS_Controller_State  Value=BMS_Controller_State.BMS_Charging  SampleTime=-1
  Driving1 : simulink/Sources/Enumerated Constant  OutDataTypeStr=Enum: BMS_Controller_State  Value=BMS_Controller_State.BMS_Fault  SampleTime=-1
  Driving2 : simulink/Sources/Enumerated Constant  OutDataTypeStr=Enum: Charging_State  Value=Charging_State.CV  SampleTime=-1
  Faults_unpacking : slrealtimeutilitieslib/Bit Unpacking  SignExtend=on  MaskBitPatterns={[7:7] [6:6] [5:5] [4:4] [3:3] [2:2] [1:1] [0:0]}  MaskPackDataType=uint8  MaskPackDataSize=[1]  MaskUnpackDataTypes={'boolean', 'boolean', 'boolean', 'boolean', 'boolean', 'boolean', 'boolean', 'boolean'}  MaskUnpackDataSizes={[1] [1] [1] [1] [1] [1] [1] [1]}
  Gain : Gain  Gain=100
  Gain1 : Gain  Gain=100
  Gain2 : Gain  Gain=100
  Multiport Switch1 : MultiPortSwitch  DataPortOrder=Zero-based contiguous  zeroidx=on  SaturateOnIntegerOverflow=off  InputSameDT=off
  Multiport Switch2 : MultiPortSwitch  DataPortOrder=Zero-based contiguous  Inputs=4  zeroidx=on  SaturateOnIntegerOverflow=off  InputSameDT=off
  Mux1 : Mux  Inputs=3
  Terminator{,1..2,4..5,7,10,13..16} (11 alike) : Terminator
  Discharge_Current_Limit : Outport
  Charge_Current_Limit : Outport  Port=2
  Charge_Current_Req : Outport  Port=3
  SOC : Outport  Port=4
  BMS_Faults : Outport  Port=5
  BMS_State : Outport  Port=6
  Charging_State : Outport  Port=7
  wires:
  CAN Unpack1/2 -> Terminator2/1
  CAN Unpack/1 -> Discharge_Current_Limit/1  "Discharge_Current_Limit"
  CAN Unpack1/1 -> Charge_Current_Req/1  "Charge_Current_Req"
  CAN Unpack1/3 -> Terminator5/1
  CAN Unpack/2 -> Charge_Current_Limit/1  "Charge_Current_Limit"
  CAN Unpack/4 -> Terminator7/1
  CAN Unpack/3 -> Terminator4/1
  ID_0x201/1 -> CAN Unpack/1
  ID_0x202/1 -> CAN Unpack1/1
  CAN Unpack2/2 -> Gain1/1
  Bus Creator/1 -> BMS_Faults/1
  Faults_unpacking/5 -> Bus Creator/5  "UnderVolt"
  CAN Unpack3/5 -> Terminator10/1
  CAN Unpack3/3 -> Multiport Switch2/1
  CAN Unpack3/2 -> Faults_unpacking/1
  Faults_unpacking/4 -> Bus Creator/4  "OverVolt"
  Faults_unpacking/3 -> Bus Creator/3  "LowTemp"
  CAN Unpack2/1 -> Gain/1
  Faults_unpacking/1 -> Bus Creator/1  "OverCurrent"
  ID_0x501/1 -> CAN Unpack2/1
  Faults_unpacking/2 -> Bus Creator/2  "HighTemp"
  CAN Unpack2/3 -> Terminator/1  "Time_0x501"
  ID_0x502/1 -> CAN Unpack3/1
  Gain/1 -> Mux1/1  "SOC_UKF"
  Gain1/1 -> Mux1/2  "SOC_EKF"
  CAN Unpack3/1 -> Gain2/1
  CAN Unpack2/4 -> Terminator1/1  "Status_0x501"
  Faults_unpacking/6 -> Terminator13/1
  Faults_unpacking/7 -> Terminator14/1
  Faults_unpacking/8 -> Terminator15/1
  CAN Unpack3/6 -> Terminator16/1
  Gain2/1 -> Mux1/3  "SOC_CC"
  Mux1/1 -> SOC/1  "SOC"
  Charging/1 -> Multiport Switch2/3
  Balancing/1 -> Multiport Switch2/2
  Driving/1 -> Multiport Switch2/4
  Driving1/1 -> Multiport Switch2/5
  Charging1/1 -> Multiport Switch1/3
  Driving2/1 -> Multiport Switch1/4
  Balancing1/1 -> Multiport Switch1/2
  CAN Unpack3/4 -> Multiport Switch1/1
  Multiport Switch1/1 -> Charging_State/1
  Multiport Switch2/1 -> BMS_State/1

== system SystemModel/BMS/HIL/Controller/PLANT-Tx/12-Cell ==
  to_Controller : Inport
  to_Controller_SRE : Inport  Port=2
  Bus Selector : BusSelector  OutputSignals=Pack_Current,Cell_Temperatures
  CAN Pack2 : canmsglib/CAN Pack  MsgList=(none)  MsgName=CAN Msg  MsgIDType=Standard (11-bit identifier)  MsgIdentifier=0x407  CANIDInput=off  MsgLength=8  Remote=off  ApplyMinMax=off  BusOutput=off  SignalInfo={ 'Cell_Temperatures_2', '0', '32', 'LE', 'single', 'Standard', '0', '1', '0', '-Inf', 'Inf'; 'Cell_Temperatures_1', '32', '32', 'LE', 'single', 'Standard', '0', '1', '0', '-Inf', 'Inf' }
      settings: LibrarySourceBlock=embeddedtargetslib/Host Communication/CAN Pack  DataFormat=manually specified signals
  CAN Pack3 : canmsglib/CAN Pack  MsgList=(none)  MsgName=CAN Msg  MsgIDType=Standard (11-bit identifier)  MsgIdentifier=0x404  CANIDInput=off  MsgLength=8  Remote=off  ApplyMinMax=off  BusOutput=off  SignalInfo={ 'Cell_Temperatures_8', '0', '32', 'LE', 'single', 'Standard', '0', '1', '0', '-Inf', 'Inf'; 'Cell_Temperatures_7', '32', '32', 'LE', 'single', 'Standard', '0', '1', '0', '-Inf', 'Inf' }
      settings: LibrarySourceBlock=embeddedtargetslib/Host Communication/CAN Pack  DataFormat=manually specified signals
  CAN Pack4 : canmsglib/CAN Pack  MsgList=(none)  MsgName=CAN Msg  MsgIDType=Standard (11-bit identifier)  MsgIdentifier=0x401  CANIDInput=off  MsgLength=5  Remote=off  ApplyMinMax=off  BusOutput=off  SignalInfo={ 'Pack_Current', '0', '32', 'LE', 'single', 'Standard', '0', '1', '0', '-Inf', 'Inf'; 'SRE', '32', '8', 'LE', 'unsigned', 'Standard', '0', '1', '0', '-Inf', 'Inf' }
      settings: LibrarySourceBlock=embeddedtargetslib/Host Communication/CAN Pack  DataFormat=manually specified signals
  CAN Pack5 : canmsglib/CAN Pack  MsgList=(none)  MsgName=CAN Msg  MsgIDType=Standard (11-bit identifier)  MsgIdentifier=0x405  CANIDInput=off  MsgLength=8  Remote=off  ApplyMinMax=off  BusOutput=off  SignalInfo={ 'Cell_Temperatures_6', '0', '32', 'LE', 'single', 'Standard', '0', '1', '0', '-Inf', 'Inf'; 'Cell_Temperatures_5', '32', '32', 'LE', 'single', 'Standard', '0', '1', '0', '-Inf', 'Inf' }
      settings: LibrarySourceBlock=embeddedtargetslib/Host Communication/CAN Pack  DataFormat=manually specified signals
  CAN Pack6 : canmsglib/CAN Pack  MsgList=(none)  MsgName=CAN Msg  MsgIDType=Standard (11-bit identifier)  MsgIdentifier=0x402  CANIDInput=off  MsgLength=8  Remote=off  ApplyMinMax=off  BusOutput=off  SignalInfo={ 'Cell_Temperatures_12', '0', '32', 'LE', 'single', 'Standard', '0', '1', '0', '-Inf', 'Inf'; 'Cell_Temperatures_11', '32', '32', 'LE', 'single', 'Standard', '0', '1', '0', '-Inf', 'Inf' }
      settings: LibrarySourceBlock=embeddedtargetslib/Host Communication/CAN Pack  DataFormat=manually specified signals
  CAN Pack7 : canmsglib/CAN Pack  MsgList=(none)  MsgName=CAN Msg  MsgIDType=Standard (11-bit identifier)  MsgIdentifier=0x403  CANIDInput=off  MsgLength=8  Remote=off  ApplyMinMax=off  BusOutput=off  SignalInfo={ 'Cell_Temperatures_10', '0', '32', 'LE', 'single', 'Standard', '0', '1', '0', '-Inf', 'Inf'; 'Cell_Temperatures_9', '32', '32', 'LE', 'single', 'Standard', '0', '1', '0', '-Inf', 'Inf' }
      settings: LibrarySourceBlock=embeddedtargetslib/Host Communication/CAN Pack  DataFormat=manually specified signals
  CAN Pack8 : canmsglib/CAN Pack  MsgList=(none)  MsgName=CAN Msg  MsgIDType=Standard (11-bit identifier)  MsgIdentifier=0x406  CANIDInput=off  MsgLength=8  Remote=off  ApplyMinMax=off  BusOutput=off  SignalInfo={ 'Cell_Temperatures_4', '0', '32', 'LE', 'single', 'Standard', '0', '1', '0', '-Inf', 'Inf'; 'Cell_Temperatures_3', '32', '32', 'LE', 'single', 'Standard', '0', '1', '0', '-Inf', 'Inf' }
      settings: LibrarySourceBlock=embeddedtargetslib/Host Communication/CAN Pack  DataFormat=manually specified signals
  CAN Write {,1..6} (7 alike) : speedgoatlib_IO611/CAN Write   moduleType=IO611  id=1  channel=2  canType=CAN (HS)  useBusIn=off  numOfMsg=1  enableInput=off  enableStatusPort=off  initValues=[611 1 -1 1 1 1 0 1 0 0]  ts=-1
      settings: SourceProductName=IO611
  Demux1 : Demux  Outputs=12
  wires:
  to_Controller/1 -> Bus Selector/1
  Bus Selector/1 -> CAN Pack4/1  "<Pack_Current>"
  Bus Selector/2 -> Demux1/1  "<Cell_Temperatures>"
  Demux1/1 -> CAN Pack6/1
  Demux1/2 -> CAN Pack6/2
  Demux1/3 -> CAN Pack7/1
  Demux1/4 -> CAN Pack7/2
  Demux1/5 -> CAN Pack3/1
  Demux1/6 -> CAN Pack3/2
  CAN Pack4/1 -> "CAN Write "/1
  CAN Pack6/1 -> CAN Write 1/1
  to_Controller_SRE/1 -> CAN Pack4/2
  CAN Pack7/1 -> CAN Write 2/1
  CAN Pack3/1 -> CAN Write 3/1
  CAN Pack2/1 -> CAN Write 6/1
  CAN Pack5/1 -> CAN Write 4/1
  CAN Pack8/1 -> CAN Write 5/1
  Demux1/7 -> CAN Pack5/1
  Demux1/8 -> CAN Pack5/2
  Demux1/9 -> CAN Pack8/1
  Demux1/10 -> CAN Pack8/2
  Demux1/11 -> CAN Pack2/1
  Demux1/12 -> CAN Pack2/2

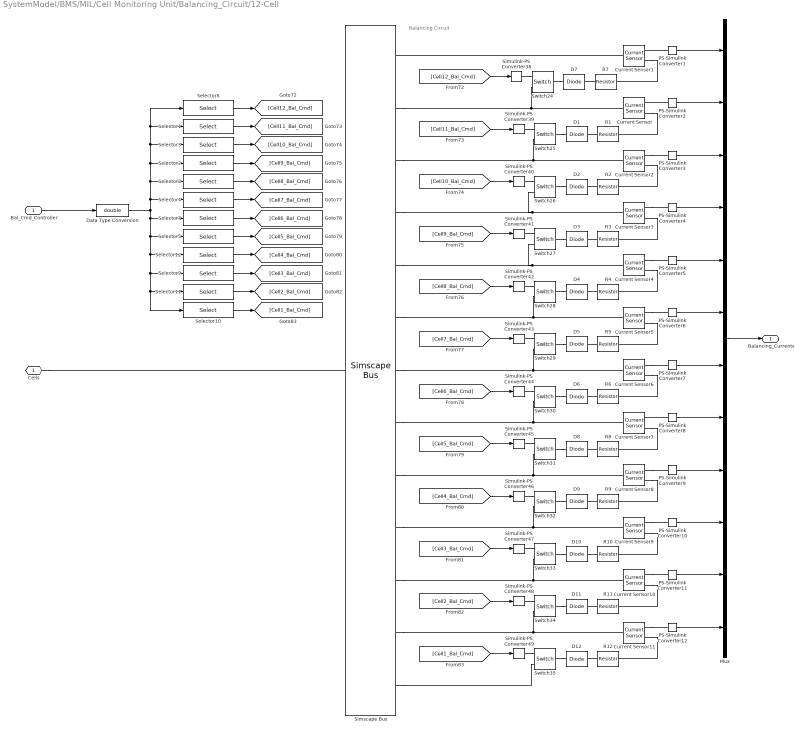
== system SystemModel/BMS/MIL/Cell Monitoring Unit/Balancing_Circuit/12-Cell ==
  note: Balancing Circuit
  Bal_Cmd_Controller : Inport
  Current Sensor{,1..11} (12 alike) : fl_lib/Electrical/Electrical Sensors/Current Sensor
  D{1..12} (12 alike) : fl_lib/Electrical/Electrical Elements/Diode  Vf=0.6 V  Ron=0.3 Ohm  Goff=1e-8 1/Ohm  i_specify=off  i_priority=High  i=0 A  i_nominal_specify=off  i_nominal_value=1  i_nominal_unit=A  v_specify=off  v_priority=None  v=0 V  v_nominal_specify=off  v_nominal_value=1  v_nominal_unit=V
      settings: LibrarySourceBlock=BatteryPack_lib/CellMonitoringUnit/D1  LogSimulationData=on
  Data Type Conversion : DataTypeConversion  OutDataTypeStr=double  SaturateOnIntegerOverflow=off  RndMeth=Floor
  Mux : Mux  Inputs=12
  PS-Simulink Converter{1..12} (12 alike) : nesl_utility/PS-Simulink Converter  PhysicalDomain=network_engine_domain  SubClassName=ps_output  LeftPortType=input  RightPortType=output  PseudoPeriodic=off  Frequencies=[]  VectorFormat=inherit  Unit=inherit  AffineConversion=off
  R{1..12} (12 alike) : fl_lib/Electrical/Electrical Elements/Resistor  R=Battery.R_bleed Ohm  i_specify=off  i_priority=None  i=0 A  i_nominal_specify=off  i_nominal_value=1  i_nominal_unit=A  v_specify=off  v_priority=None  v=0 V  v_nominal_specify=off  v_nominal_value=1  v_nominal_unit=V
      settings: LibrarySourceBlock=BatteryPack_lib/CellMonitoringUnit/R1  LogSimulationData=on
  Selector1 : Selector  IndexOptions=Index vector (dialog)  Indices=2  OutputSizes=1
  Selector10 : Selector  IndexOptions=Index vector (dialog)  Indices=12  OutputSizes=1
  Selector11 : Selector  IndexOptions=Index vector (dialog)  Indices=11  OutputSizes=1
  Selector12 : Selector  IndexOptions=Index vector (dialog)  Indices=9  OutputSizes=1
  Selector2 : Selector  IndexOptions=Index vector (dialog)  Indices=4  OutputSizes=1
  Selector3 : Selector  IndexOptions=Index vector (dialog)  Indices=3  OutputSizes=1
  Selector4 : Selector  IndexOptions=Index vector (dialog)  Indices=6  OutputSizes=1
  Selector5 : Selector  IndexOptions=Index vector (dialog)  Indices=8  OutputSizes=1
  Selector6 : Selector  IndexOptions=Index vector (dialog)  Indices=1  OutputSizes=1
  Selector7 : Selector  IndexOptions=Index vector (dialog)  Indices=7  OutputSizes=1
  Selector8 : Selector  IndexOptions=Index vector (dialog)  Indices=5  OutputSizes=1
  Selector9 : Selector  IndexOptions=Index vector (dialog)  Indices=10  OutputSizes=1
  Simscape Bus : SimscapeBus  HierarchyStrings=Cell12_P;Cell11_P;Cell10_P;Cell9_P;Cell8_P;Cell7_P;Cell6_P;Cell5_P;Cell4_P;Cell3_P;Cell2_P;Cell1_P;Cell1_N
  Simulink-PS Converter{38..49} (12 alike) : nesl_utility/Simulink-PS Converter  PhysicalDomain=network_engine_domain  SubClassName=ps_input  LeftPortType=input  RightPortType=output  PseudoPeriodic=off  Frequencies=[]  NoiseDistribution=none  NoiseParameters=[]  Unit=1  AffineConversion=off  FilteringAndDerivatives=zero  SimscapeFilterOrder=1  InputFilterTimeConstant=0.001  UdotUserProvided=1
      settings: LibrarySourceBlock=|
      | BatteryPack_lib/CellMonitoringUnit/Simulink-PS
      | Converter3
  Switch{24..35} (12 alike) : fl_lib/Electrical/Electrical Elements/Switch  R_closed=0.01 Ohm  G_open=1e-8 1/Ohm  Threshold=0  i_specify=off  i_priority=None  i=0 A  i_nominal_specify=off  i_nominal_value=1  i_nominal_unit=A  v_specify=off  v_priority=None  v=0 V  v_nominal_specify=off  v_nominal_value=1  v_nominal_unit=V
      settings: LibrarySourceBlock=BatteryPack_lib/CellMonitoringUnit/Switch
  Cells : PMIOPort  Side=Left
  Balancing_Currents : Outport
  wires:
  [Cell3_Bal_Cmd] -> Simulink-PS Converter47/1
  [Cell4_Bal_Cmd] -> Simulink-PS Converter46/1
  [Cell2_Bal_Cmd] -> Simulink-PS Converter48/1
  [Cell9_Bal_Cmd] -> Simulink-PS Converter41/1
  [Cell12_Bal_Cmd] -> Simulink-PS Converter38/1
  [Cell6_Bal_Cmd] -> Simulink-PS Converter44/1
  [Cell11_Bal_Cmd] -> Simulink-PS Converter39/1
  [Cell1_Bal_Cmd] -> Simulink-PS Converter49/1
  [Cell10_Bal_Cmd] -> Simulink-PS Converter40/1
  [Cell8_Bal_Cmd] -> Simulink-PS Converter42/1
  [Cell7_Bal_Cmd] -> Simulink-PS Converter43/1
  [Cell5_Bal_Cmd] -> Simulink-PS Converter45/1
  Selector11/1 -> [Cell2_Bal_Cmd]
  Selector12/1 -> [Cell4_Bal_Cmd]
  Selector3/1 -> [Cell10_Bal_Cmd]
  Selector9/1 -> [Cell3_Bal_Cmd]
  Selector1/1 -> [Cell11_Bal_Cmd]
  Selector4/1 -> [Cell7_Bal_Cmd]
  Selector8/1 -> [Cell8_Bal_Cmd]
  Selector6/1 -> [Cell12_Bal_Cmd]
  Selector7/1 -> [Cell6_Bal_Cmd]
  Selector5/1 -> [Cell5_Bal_Cmd]
  Selector10/1 -> [Cell1_Bal_Cmd]
  Selector2/1 -> [Cell9_Bal_Cmd]
  Data Type Conversion/1 -> Selector4/1, Selector8/1, Selector2/1, Selector3/1, Selector1/1, Selector6/1, Selector7/1, Selector5/1, Selector12/1, Selector9/1, Selector11/1, Selector10/1
  Bal_Cmd_Controller/1 -> Data Type Conversion/1
  PS-Simulink Converter1/1 -> Mux/1
  PS-Simulink Converter12/1 -> Mux/12
  PS-Simulink Converter2/1 -> Mux/2
  PS-Simulink Converter3/1 -> Mux/3
  PS-Simulink Converter4/1 -> Mux/4
  PS-Simulink Converter5/1 -> Mux/5
  PS-Simulink Converter6/1 -> Mux/6
  PS-Simulink Converter7/1 -> Mux/7
  PS-Simulink Converter8/1 -> Mux/8
  PS-Simulink Converter9/1 -> Mux/9
  PS-Simulink Converter10/1 -> Mux/10
  PS-Simulink Converter11/1 -> Mux/11
  Mux/1 -> Balancing_Currents/1
  connections:
  Simscape Bus/LConn6 -- Current Sensor5/LConn1 -- Switch28/RConn2
  Simscape Bus/LConn3 -- Current Sensor2/LConn1 -- Switch25/RConn2
  Simscape Bus/LConn5 -- Current Sensor4/LConn1 -- Switch27/RConn2
  Simscape Bus/LConn12 -- Current Sensor11/LConn1 -- Switch34/RConn2
  Simscape Bus/LConn4 -- Current Sensor3/LConn1 -- Switch26/RConn2
  Simscape Bus/LConn10 -- Current Sensor9/LConn1 -- Switch32/RConn2
  Simscape Bus/LConn8 -- Current Sensor7/LConn1 -- Switch30/RConn2
  Simscape Bus/LConn2 -- Current Sensor/LConn1 -- Switch24/RConn2
  Simscape Bus/LConn9 -- Current Sensor8/LConn1 -- Switch31/RConn2
  Simscape Bus/LConn7 -- Current Sensor6/LConn1 -- Switch29/RConn2
  Simscape Bus/LConn11 -- Current Sensor10/LConn1 -- Switch33/RConn2
  Simulink-PS Converter38/RConn1 -- Switch24/RConn1
  R4/RConn1 -- D4/LConn1
  Simulink-PS Converter48/RConn1 -- Switch34/RConn1
  R7/RConn1 -- D7/LConn1
  R8/RConn1 -- D8/LConn1
  Switch25/LConn1 -- D1/RConn1
  R6/RConn1 -- D6/LConn1
  R10/RConn1 -- D10/LConn1
  R12/RConn1 -- D12/LConn1
  Simulink-PS Converter49/RConn1 -- Switch35/RConn1
  R11/RConn1 -- D11/LConn1
  Switch30/LConn1 -- D6/RConn1
  Simulink-PS Converter41/RConn1 -- Switch27/RConn1
  Switch32/LConn1 -- D9/RConn1
  Switch31/LConn1 -- D8/RConn1
  Simulink-PS Converter39/RConn1 -- Switch25/RConn1
  Switch24/LConn1 -- D7/RConn1
  Simulink-PS Converter47/RConn1 -- Switch33/RConn1
  Simulink-PS Converter46/RConn1 -- Switch32/RConn1
  Switch35/LConn1 -- D12/RConn1
  Switch29/LConn1 -- D5/RConn1
  R2/RConn1 -- D2/LConn1
  Simulink-PS Converter44/RConn1 -- Switch30/RConn1
  Switch27/LConn1 -- D3/RConn1
  Switch28/LConn1 -- D4/RConn1
  Simulink-PS Converter43/RConn1 -- Switch29/RConn1
  Simulink-PS Converter45/RConn1 -- Switch31/RConn1
  R3/RConn1 -- D3/LConn1
  R9/RConn1 -- D9/LConn1
  Simulink-PS Converter42/RConn1 -- Switch28/RConn1
  Switch26/LConn1 -- D2/RConn1
  Simulink-PS Converter40/RConn1 -- Switch26/RConn1
  R5/RConn1 -- D5/LConn1
  Switch33/LConn1 -- D10/RConn1
  Switch34/LConn1 -- D11/RConn1
  R1/RConn1 -- D1/LConn1
  Simscape Bus/LConn13 -- Switch35/RConn2
  Cells/RConn1 -- Simscape Bus/RConn1
  Current Sensor1/LConn1 -- Simscape Bus/LConn1
  Current Sensor1/RConn2 -- R7/LConn1
  Current Sensor2/RConn2 -- R2/LConn1
  Current Sensor3/RConn2 -- R3/LConn1
  Current Sensor4/RConn2 -- R4/LConn1
  Current Sensor5/RConn2 -- R5/LConn1
  Current Sensor6/RConn2 -- R6/LConn1
  Current Sensor7/RConn2 -- R8/LConn1
  Current Sensor8/RConn2 -- R9/LConn1
  Current Sensor9/RConn2 -- R10/LConn1
  Current Sensor10/RConn2 -- R11/LConn1
  Current Sensor11/RConn2 -- R12/LConn1
  Current Sensor/RConn2 -- R1/LConn1
  PS-Simulink Converter1/LConn1 -- Current Sensor1/RConn1
  PS-Simulink Converter2/LConn1 -- Current Sensor/RConn1
  Current Sensor2/RConn1 -- PS-Simulink Converter3/LConn1
  Current Sensor3/RConn1 -- PS-Simulink Converter4/LConn1
  PS-Simulink Converter8/LConn1 -- Current Sensor7/RConn1
  Current Sensor6/RConn1 -- PS-Simulink Converter7/LConn1
  Current Sensor5/RConn1 -- PS-Simulink Converter6/LConn1
  Current Sensor4/RConn1 -- PS-Simulink Converter5/LConn1
  Current Sensor8/RConn1 -- PS-Simulink Converter9/LConn1
  Current Sensor9/RConn1 -- PS-Simulink Converter10/LConn1
  Current Sensor10/RConn1 -- PS-Simulink Converter11/LConn1
  Current Sensor11/RConn1 -- PS-Simulink Converter12/LConn1

== system SystemModel/BMS/MIL/Controller/Current Calculations/Charge_Current_Limit_Calc ==
  MaxCellVolt : Inport
  MinCellTemp : Inport  Port=2
  MaxCellTemp : Inport  Port=3
  Divide1 : Product  Inputs=*/
  HighTempChrgCurrentLim : Lookup_n-D  NumberOfTableDimensions=1  BreakpointsForDimension1=273.15+[-30:1:70]  Table=50*(1-tanh(273.15+[-30:1:70]-273.15-50))/2  InternalRulePriority=Speed  RndMeth=Simplest
  InternalCellResistance : Constant  Value=single(max(max(Battery(1).R0_LUT)))  OutDataTypeStr=single  SampleTime=-1
  LowTempChrgCurrentLim : Lookup_n-D  NumberOfTableDimensions=1  BreakpointsForDimension1=273.15+[-30:1:70]  Table=50*(1+tanh(273.15+[-30:1:70]-(273.15)))/2  InternalRulePriority=Speed  RndMeth=Simplest
  MinMax2 : MinMax  Inputs=3
  OverVoltageLimit : Constant  Value=OverCellVoltageLimit  OutDataTypeStr=single  SampleTime=-1
  Subtract1 : Sum  Inputs=+-
  Charge_Current_Limit : Outport  VectorParamsAs1DForOutWhenUnconnected=off
  wires:
  OverVoltageLimit/1 -> Subtract1/1
  MinMax2/1 -> Charge_Current_Limit/1  "ChargeCurrentLimit"
  MaxCellVolt/1 -> Subtract1/2
  Subtract1/1 -> Divide1/1
  Divide1/1 -> MinMax2/1
  InternalCellResistance/1 -> Divide1/2
  MinCellTemp/1 -> LowTempChrgCurrentLim/1
  MaxCellTemp/1 -> HighTempChrgCurrentLim/1
  HighTempChrgCurrentLim/1 -> MinMax2/3
  LowTempChrgCurrentLim/1 -> MinMax2/2
